simulink model "Model_IEEE_39Bus_GFM_80pct"  (R2024b)
settings: Solver=FixedStepAuto  StartTime=0  StopTime=5  FixedStep=Ts  RelTol=1e-3
values from neighbouring files (symbols this model uses):
  ApparatusDiscreDamping =     [Data_IEEE_39Bus_GFM_100pct.mat]    (also in Data_IEEE_39Bus_GFM_20pct.mat; Data_IEEE_39Bus_GFM_40pct.mat; Data_IEEE_39Bus_GFM_60pct.mat; Data_IEEE_39Bus_GFM_80pct.mat)
  ApparatusPara =     [Data_IEEE_39Bus_GFM_100pct.mat]    (also in Data_IEEE_39Bus_GFM_20pct.mat; Data_IEEE_39Bus_GFM_40pct.mat; Data_IEEE_39Bus_GFM_60pct.mat; Data_IEEE_39Bus_GFM_80pct.mat)
  ApparatusPowerFlow =     [Data_IEEE_39Bus_GFM_100pct.mat]    (also in Data_IEEE_39Bus_GFM_20pct.mat; Data_IEEE_39Bus_GFM_40pct.mat; Data_IEEE_39Bus_GFM_60pct.mat; Data_IEEE_39Bus_GFM_80pct.mat)
  ApparatusType =     [Data_IEEE_39Bus_GFM_100pct.mat]    (also in Data_IEEE_39Bus_GFM_20pct.mat; Data_IEEE_39Bus_GFM_40pct.mat; Data_IEEE_39Bus_GFM_60pct.mat; Data_IEEE_39Bus_GFM_80pct.mat)
  Fbase = 60    [Data_IEEE_39Bus_GFM_100pct.mat]    (also in Data_IEEE_39Bus_GFM_20pct.mat; Data_IEEE_39Bus_GFM_40pct.mat; Data_IEEE_39Bus_GFM_60pct.mat; Data_IEEE_39Bus_GFM_80pct.mat)
  OtherInputs =     [Data_IEEE_39Bus_GFM_100pct.mat]    (also in Data_IEEE_39Bus_GFM_20pct.mat; Data_IEEE_39Bus_GFM_40pct.mat; Data_IEEE_39Bus_GFM_60pct.mat; Data_IEEE_39Bus_GFM_80pct.mat)
  Sbase = 1    [Data_IEEE_39Bus_GFM_100pct.mat]    (also in Data_IEEE_39Bus_GFM_20pct.mat; Data_IEEE_39Bus_GFM_40pct.mat; Data_IEEE_39Bus_GFM_60pct.mat; Data_IEEE_39Bus_GFM_80pct.mat)
  Ts = 3.33333333333e-05    [Data_IEEE_39Bus_GFM_100pct.mat]    (also in Data_IEEE_39Bus_GFM_20pct.mat; Data_IEEE_39Bus_GFM_40pct.mat; Data_IEEE_39Bus_GFM_60pct.mat; Data_IEEE_39Bus_GFM_80pct.mat)
  Vbase = 1    [Data_IEEE_39Bus_GFM_100pct.mat]    (also in Data_IEEE_39Bus_GFM_20pct.mat; Data_IEEE_39Bus_GFM_40pct.mat; Data_IEEE_39Bus_GFM_60pct.mat; Data_IEEE_39Bus_GFM_80pct.mat)
  Wbase = 376.991118431    [Data_IEEE_39Bus_GFM_100pct.mat]    (also in Data_IEEE_39Bus_GFM_20pct.mat; Data_IEEE_39Bus_GFM_40pct.mat; Data_IEEE_39Bus_GFM_60pct.mat; Data_IEEE_39Bus_GFM_80pct.mat)
  x_e =     [Data_IEEE_39Bus_GFM_100pct.mat]    (also in Data_IEEE_39Bus_GFM_20pct.mat; Data_IEEE_39Bus_GFM_40pct.mat; Data_IEEE_39Bus_GFM_60pct.mat; Data_IEEE_39Bus_GFM_80pct.mat)
  Ybase = 1    [Data_IEEE_39Bus_GFM_100pct.mat]    (also in Data_IEEE_39Bus_GFM_20pct.mat; Data_IEEE_39Bus_GFM_40pct.mat; Data_IEEE_39Bus_GFM_60pct.mat; Data_IEEE_39Bus_GFM_80pct.mat)
  Zbase = 1    [Data_IEEE_39Bus_GFM_100pct.mat]    (also in Data_IEEE_39Bus_GFM_20pct.mat; Data_IEEE_39Bus_GFM_40pct.mat; Data_IEEE_39Bus_GFM_60pct.mat; Data_IEEE_39Bus_GFM_80pct.mat)
libraries: SimplusGT x49, spsThreePhaseSeriesRLCBranchLib x46, spsGroundLib x41, spsThreePhaseParallelRLCBranchLib x31, spsThreePhaseTransformerTwoWindingsLib x11, spspowerguiLib x1
settings Model: Creator=皮蛋蛋挞  LastModifiedBy=皮蛋蛋挞

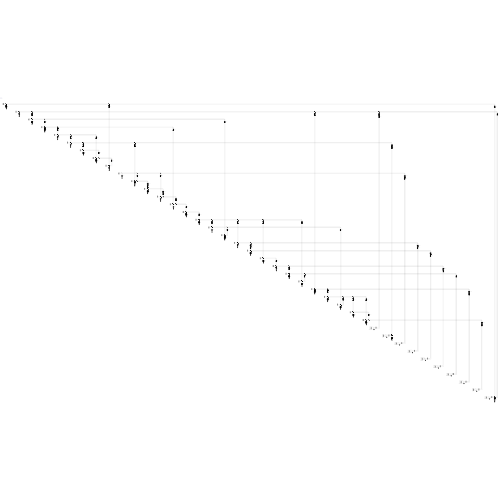
[thumbnail: Simulink's stored preview of the top-level diagram]
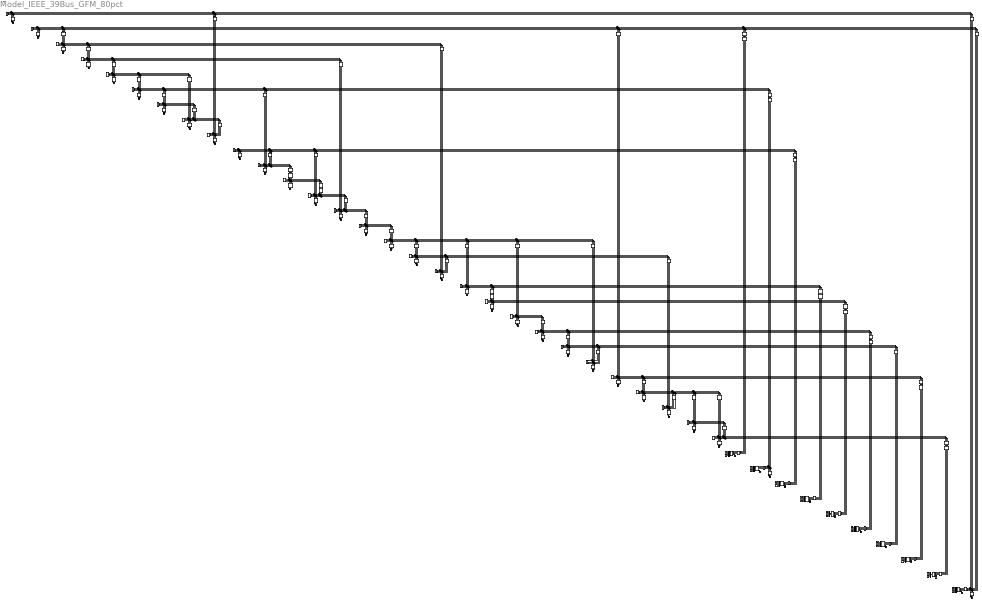
== system Model_IEEE_39Bus_GFM_80pct ==
  B-GND{1,4,9,12,15,18,22,24,26..27,31,33,35,37,39,41,46,49..50,53,55,57,60,63..64,67,71..72,74,76..77} (31 alike) : spsGroundLib/Ground  LConnTagsString=a
  Branch1-1 : spsThreePhaseParallelRLCBranchLib/Three-Phase Parallel RLC Branch  LConnTagsString=A|B|C  RConnTagsString=A|B|C  BranchType=RLC  Resistance=(0.096096)*Zbase  Inductance=(0.42436)*Zbase/Wbase  Capacitance=(0.975)*Ybase/Wbase  Measurements=None
  Branch1-39 : spsThreePhaseSeriesRLCBranchLib/Three-Phase Series RLC Branch  LConnTagsString=A|B|C  RConnTagsString=A|B|C  BranchType=RL  Resistance=(0.001)*Zbase  Inductance=(0.025)*Zbase/Wbase  Capacitance=1e-6  Measurements=None
  Branch1-9 : spsThreePhaseSeriesRLCBranchLib/Three-Phase Series RLC Branch  LConnTagsString=A|B|C  RConnTagsString=A|B|C  BranchType=RL  Resistance=(0.001)*Zbase  Inductance=(0.025)*Zbase/Wbase  Capacitance=1e-6  Measurements=None
  Branch10-10 : spsThreePhaseParallelRLCBranchLib/Three-Phase Parallel RLC Branch  LConnTagsString=A|B|C  RConnTagsString=A|B|C  BranchType=C  Resistance=(Inf)*Zbase  Inductance=(Inf)*Zbase/Wbase  Capacitance=(0.0729)*Ybase/Wbase  Measurements=None
  Branch10-11 : spsThreePhaseSeriesRLCBranchLib/Three-Phase Series RLC Branch  LConnTagsString=A|B|C  RConnTagsString=A|B|C  BranchType=RL  Resistance=(0.0004)*Zbase  Inductance=(0.0043)*Zbase/Wbase  Capacitance=1e-6  Measurements=None
  Branch10-13 : spsThreePhaseSeriesRLCBranchLib/Three-Phase Series RLC Branch  LConnTagsString=A|B|C  RConnTagsString=A|B|C  BranchType=RL  Resistance=(0.0004)*Zbase  Inductance=(0.0043)*Zbase/Wbase  Capacitance=1e-6  Measurements=None
  Branch10-32 : spsThreePhaseSeriesRLCBranchLib/Three-Phase Series RLC Branch  LConnTagsString=A|B|C  RConnTagsString=A|B|C  BranchType=RL  Resistance=(0.001)*Zbase  Inductance=(0.02)*Zbase/Wbase  Capacitance=1e-6  Measurements=None
  Branch11-11 : spsThreePhaseParallelRLCBranchLib/Three-Phase Parallel RLC Branch  LConnTagsString=A|B|C  RConnTagsString=A|B|C  BranchType=C  Resistance=(Inf)*Zbase  Inductance=(Inf)*Zbase/Wbase  Capacitance=(0.1059)*Ybase/Wbase  Measurements=None
  Branch11-12 : spsThreePhaseSeriesRLCBranchLib/Three-Phase Series RLC Branch  LConnTagsString=A|B|C  RConnTagsString=A|B|C  BranchType=RL  Resistance=(0.0016193)*Zbase  Inductance=(0.044024)*Zbase/Wbase  Capacitance=1e-6  Measurements=None
  Branch12-12 : spsThreePhaseParallelRLCBranchLib/Three-Phase Parallel RLC Branch  LConnTagsString=A|B|C  RConnTagsString=A|B|C  BranchType=RL  Resistance=(13.5473)*Zbase  Inductance=(1.1546)*Zbase/Wbase  Capacitance=(0)*Ybase/Wbase  Measurements=None
  Branch12-13 : spsThreePhaseSeriesRLCBranchLib/Three-Phase Series RLC Branch  LConnTagsString=A|B|C  RConnTagsString=A|B|C  BranchType=RL  Resistance=(0.0016)*Zbase  Inductance=(0.0435)*Zbase/Wbase  Capacitance=1e-6  Measurements=None
  Branch13-13 : spsThreePhaseParallelRLCBranchLib/Three-Phase Parallel RLC Branch  LConnTagsString=A|B|C  RConnTagsString=A|B|C  BranchType=C  Resistance=(Inf)*Zbase  Inductance=(Inf)*Zbase/Wbase  Capacitance=(0.1226)*Ybase/Wbase  Measurements=None
  Branch13-14 : spsThreePhaseSeriesRLCBranchLib/Three-Phase Series RLC Branch  LConnTagsString=A|B|C  RConnTagsString=A|B|C  BranchType=RL  Resistance=(0.0009)*Zbase  Inductance=(0.0101)*Zbase/Wbase  Capacitance=1e-6  Measurements=None
  Branch14-14 : spsThreePhaseParallelRLCBranchLib/Three-Phase Parallel RLC Branch  LConnTagsString=A|B|C  RConnTagsString=A|B|C  BranchType=C  Resistance=(Inf)*Zbase  Inductance=(Inf)*Zbase/Wbase  Capacitance=(0.33825)*Ybase/Wbase  Measurements=None
  Branch14-15 : spsThreePhaseSeriesRLCBranchLib/Three-Phase Series RLC Branch  LConnTagsString=A|B|C  RConnTagsString=A|B|C  BranchType=RL  Resistance=(0.0018)*Zbase  Inductance=(0.0217)*Zbase/Wbase  Capacitance=1e-6  Measurements=None
  Branch15-15 : spsThreePhaseParallelRLCBranchLib/Three-Phase Parallel RLC Branch  LConnTagsString=A|B|C  RConnTagsString=A|B|C  BranchType=RLC  Resistance=(0.32386)*Zbase  Inductance=(0.67736)*Zbase/Wbase  Capacitance=(0.2685)*Ybase/Wbase  Measurements=None
  Branch15-16 : spsThreePhaseSeriesRLCBranchLib/Three-Phase Series RLC Branch  LConnTagsString=A|B|C  RConnTagsString=A|B|C  BranchType=RL  Resistance=(0.0009)*Zbase  Inductance=(0.0094)*Zbase/Wbase  Capacitance=1e-6  Measurements=None
  Branch16-16 : spsThreePhaseParallelRLCBranchLib/Three-Phase Parallel RLC Branch  LConnTagsString=A|B|C  RConnTagsString=A|B|C  BranchType=RLC  Resistance=(0.3242)*Zbase  Inductance=(3.3023)*Zbase/Wbase  Capacitance=(0.466)*Ybase/Wbase  Measurements=None
  Branch16-17 : spsThreePhaseSeriesRLCBranchLib/Three-Phase Series RLC Branch  LConnTagsString=A|B|C  RConnTagsString=A|B|C  BranchType=RL  Resistance=(0.0007)*Zbase  Inductance=(0.0089)*Zbase/Wbase  Capacitance=1e-6  Measurements=None
  Branch16-19 : spsThreePhaseSeriesRLCBranchLib/Three-Phase Series RLC Branch  LConnTagsString=A|B|C  RConnTagsString=A|B|C  BranchType=RL  Resistance=(0.0016)*Zbase  Inductance=(0.0195)*Zbase/Wbase  Capacitance=1e-6  Measurements=None
  Branch16-21 : spsThreePhaseSeriesRLCBranchLib/Three-Phase Series RLC Branch  LConnTagsString=A|B|C  RConnTagsString=A|B|C  BranchType=RL  Resistance=(0.0008)*Zbase  Inductance=(0.0135)*Zbase/Wbase  Capacitance=1e-6  Measurements=None
  Branch16-24 : spsThreePhaseSeriesRLCBranchLib/Three-Phase Series RLC Branch  LConnTagsString=A|B|C  RConnTagsString=A|B|C  BranchType=RL  Resistance=(0.0003)*Zbase  Inductance=(0.0059)*Zbase/Wbase  Capacitance=1e-6  Measurements=None
  Branch17-17 : spsThreePhaseParallelRLCBranchLib/Three-Phase Parallel RLC Branch  LConnTagsString=A|B|C  RConnTagsString=A|B|C  BranchType=C  Resistance=(Inf)*Zbase  Inductance=(Inf)*Zbase/Wbase  Capacitance=(0.29385)*Ybase/Wbase  Measurements=None
  Branch17-18 : spsThreePhaseSeriesRLCBranchLib/Three-Phase Series RLC Branch  LConnTagsString=A|B|C  RConnTagsString=A|B|C  BranchType=RL  Resistance=(0.0007)*Zbase  Inductance=(0.0082)*Zbase/Wbase  Capacitance=1e-6  Measurements=None
  Branch17-27 : spsThreePhaseSeriesRLCBranchLib/Three-Phase Series RLC Branch  LConnTagsString=A|B|C  RConnTagsString=A|B|C  BranchType=RL  Resistance=(0.0013)*Zbase  Inductance=(0.0173)*Zbase/Wbase  Capacitance=1e-6  Measurements=None
  Branch18-18 : spsThreePhaseParallelRLCBranchLib/Three-Phase Parallel RLC Branch  LConnTagsString=A|B|C  RConnTagsString=A|B|C  BranchType=RLC  Resistance=(0.6754)*Zbase  Inductance=(3.5571)*Zbase/Wbase  Capacitance=(0.17285)*Ybase/Wbase  Measurements=None
  Branch19-19 : spsThreePhaseParallelRLCBranchLib/Three-Phase Parallel RLC Branch  LConnTagsString=A|B|C  RConnTagsString=A|B|C  BranchType=C  Resistance=(Inf)*Zbase  Inductance=(Inf)*Zbase/Wbase  Capacitance=(0.152)*Ybase/Wbase  Measurements=None
  Branch19-20 : spsThreePhaseSeriesRLCBranchLib/Three-Phase Series RLC Branch  LConnTagsString=A|B|C  RConnTagsString=A|B|C  BranchType=RL  Resistance=(0.0007)*Zbase  Inductance=(0.0138)*Zbase/Wbase  Capacitance=1e-6  Measurements=None
  Branch19-33 : spsThreePhaseSeriesRLCBranchLib/Three-Phase Series RLC Branch  LConnTagsString=A|B|C  RConnTagsString=A|B|C  BranchType=RL  Resistance=(0.0007)*Zbase  Inductance=(0.0142)*Zbase/Wbase  Capacitance=1e-6  Measurements=None
  Branch2-2 : spsThreePhaseParallelRLCBranchLib/Three-Phase Parallel RLC Branch  LConnTagsString=A|B|C  RConnTagsString=A|B|C  BranchType=C  Resistance=(Inf)*Zbase  Inductance=(Inf)*Zbase/Wbase  Capacitance=(0.55095)*Ybase/Wbase  Measurements=None
  Branch2-25 : spsThreePhaseSeriesRLCBranchLib/Three-Phase Series RLC Branch  LConnTagsString=A|B|C  RConnTagsString=A|B|C  BranchType=RL  Resistance=(0.007)*Zbase  Inductance=(0.0086)*Zbase/Wbase  Capacitance=1e-6  Measurements=None
  Branch2-3 : spsThreePhaseSeriesRLCBranchLib/Three-Phase Series RLC Branch  LConnTagsString=A|B|C  RConnTagsString=A|B|C  BranchType=RL  Resistance=(0.0013)*Zbase  Inductance=(0.0151)*Zbase/Wbase  Capacitance=1e-6  Measurements=None
  Branch2-30 : spsThreePhaseSeriesRLCBranchLib/Three-Phase Series RLC Branch  LConnTagsString=A|B|C  RConnTagsString=A|B|C  BranchType=RL  Resistance=(0.001)*Zbase  Inductance=(0.0181)*Zbase/Wbase  Capacitance=1e-6  Measurements=None
  Branch2-39 : spsThreePhaseSeriesRLCBranchLib/Three-Phase Series RLC Branch  LConnTagsString=A|B|C  RConnTagsString=A|B|C  BranchType=RL  Resistance=(0.0035)*Zbase  Inductance=(0.0411)*Zbase/Wbase  Capacitance=1e-6  Measurements=None
  Branch20-20 : spsThreePhaseParallelRLCBranchLib/Three-Phase Parallel RLC Branch  LConnTagsString=A|B|C  RConnTagsString=A|B|C  BranchType=RL  Resistance=(0.1565)*Zbase  Inductance=(0.9542)*Zbase/Wbase  Capacitance=(0)*Ybase/Wbase  Measurements=None
  Branch20-34 : spsThreePhaseSeriesRLCBranchLib/Three-Phase Series RLC Branch  LConnTagsString=A|B|C  RConnTagsString=A|B|C  BranchType=RL  Resistance=(0.0009)*Zbase  Inductance=(0.018)*Zbase/Wbase  Capacitance=1e-6  Measurements=None
  Branch21-21 : spsThreePhaseParallelRLCBranchLib/Three-Phase Parallel RLC Branch  LConnTagsString=A|B|C  RConnTagsString=A|B|C  BranchType=RLC  Resistance=(0.38793)*Zbase  Inductance=(0.92428)*Zbase/Wbase  Capacitance=(0.25565)*Ybase/Wbase  Measurements=None
  Branch21-22 : spsThreePhaseSeriesRLCBranchLib/Three-Phase Series RLC Branch  LConnTagsString=A|B|C  RConnTagsString=A|B|C  BranchType=RL  Resistance=(0.0008)*Zbase  Inductance=(0.014)*Zbase/Wbase  Capacitance=1e-6  Measurements=None
  Branch22-22 : spsThreePhaseParallelRLCBranchLib/Three-Phase Parallel RLC Branch  LConnTagsString=A|B|C  RConnTagsString=A|B|C  BranchType=C  Resistance=(Inf)*Zbase  Inductance=(Inf)*Zbase/Wbase  Capacitance=(0.22055)*Ybase/Wbase  Measurements=None
  Branch22-23 : spsThreePhaseSeriesRLCBranchLib/Three-Phase Series RLC Branch  LConnTagsString=A|B|C  RConnTagsString=A|B|C  BranchType=RL  Resistance=(0.0006)*Zbase  Inductance=(0.0096)*Zbase/Wbase  Capacitance=1e-6  Measurements=None
  Branch22-35 : spsThreePhaseSeriesRLCBranchLib/Three-Phase Series RLC Branch  LConnTagsString=A|B|C  RConnTagsString=A|B|C  BranchType=RL  Resistance=(0.001)*Zbase  Inductance=(0.0143)*Zbase/Wbase  Capacitance=1e-6  Measurements=None
  Branch23-23 : spsThreePhaseParallelRLCBranchLib/Three-Phase Parallel RLC Branch  LConnTagsString=A|B|C  RConnTagsString=A|B|C  BranchType=RLC  Resistance=(0.43976)*Zbase  Inductance=(1.2865)*Zbase/Wbase  Capacitance=(0.2728)*Ybase/Wbase  Measurements=None
  Branch23-24 : spsThreePhaseSeriesRLCBranchLib/Three-Phase Series RLC Branch  LConnTagsString=A|B|C  RConnTagsString=A|B|C  BranchType=RL  Resistance=(0.0022)*Zbase  Inductance=(0.035)*Zbase/Wbase  Capacitance=1e-6  Measurements=None
  Branch23-36 : spsThreePhaseSeriesRLCBranchLib/Three-Phase Series RLC Branch  LConnTagsString=A|B|C  RConnTagsString=A|B|C  BranchType=RL  Resistance=(0.0005)*Zbase  Inductance=(0.0272)*Zbase/Wbase  Capacitance=1e-6  Measurements=None
  Branch24-24 : spsThreePhaseParallelRLCBranchLib/Three-Phase Parallel RLC Branch  LConnTagsString=A|B|C  RConnTagsString=A|B|C  BranchType=RC  Resistance=(0.3491)*Zbase  Inductance=(Inf)*Zbase/Wbase  Capacitance=(1.0685)*Ybase/Wbase  Measurements=None
  Branch25-25 : spsThreePhaseParallelRLCBranchLib/Three-Phase Parallel RLC Branch  LConnTagsString=A|B|C  RConnTagsString=A|B|C  BranchType=RLC  Resistance=(0.49976)*Zbase  Inductance=(2.3717)*Zbase/Wbase  Capacitance=(0.3295)*Ybase/Wbase  Measurements=None
  Branch25-26 : spsThreePhaseSeriesRLCBranchLib/Three-Phase Series RLC Branch  LConnTagsString=A|B|C  RConnTagsString=A|B|C  BranchType=RL  Resistance=(0.0032)*Zbase  Inductance=(0.0323)*Zbase/Wbase  Capacitance=1e-6  Measurements=None
  Branch25-37 : spsThreePhaseSeriesRLCBranchLib/Three-Phase Series RLC Branch  LConnTagsString=A|B|C  RConnTagsString=A|B|C  BranchType=RL  Resistance=(0.0006)*Zbase  Inductance=(0.0232)*Zbase/Wbase  Capacitance=1e-6  Measurements=None
  Branch26-26 : spsThreePhaseParallelRLCBranchLib/Three-Phase Parallel RLC Branch  LConnTagsString=A|B|C  RConnTagsString=A|B|C  BranchType=RLC  Resistance=(0.7975)*Zbase  Inductance=(6.5207)*Zbase/Wbase  Capacitance=(1.2809)*Ybase/Wbase  Measurements=None
  Branch26-27 : spsThreePhaseSeriesRLCBranchLib/Three-Phase Series RLC Branch  LConnTagsString=A|B|C  RConnTagsString=A|B|C  BranchType=RL  Resistance=(0.0014)*Zbase  Inductance=(0.0147)*Zbase/Wbase  Capacitance=1e-6  Measurements=None
  Branch26-28 : spsThreePhaseSeriesRLCBranchLib/Three-Phase Series RLC Branch  LConnTagsString=A|B|C  RConnTagsString=A|B|C  BranchType=RL  Resistance=(0.0043)*Zbase  Inductance=(0.0474)*Zbase/Wbase  Capacitance=1e-6  Measurements=None
  Branch26-29 : spsThreePhaseSeriesRLCBranchLib/Three-Phase Series RLC Branch  LConnTagsString=A|B|C  RConnTagsString=A|B|C  BranchType=RL  Resistance=(0.0057)*Zbase  Inductance=(0.0625)*Zbase/Wbase  Capacitance=1e-6  Measurements=None
  Branch27-27 : spsThreePhaseParallelRLCBranchLib/Three-Phase Parallel RLC Branch  LConnTagsString=A|B|C  RConnTagsString=A|B|C  BranchType=RLC  Resistance=(0.38408)*Zbase  Inductance=(1.4295)*Zbase/Wbase  Capacitance=(0.2806)*Ybase/Wbase  Measurements=None
  Branch28-28 : spsThreePhaseParallelRLCBranchLib/Three-Phase Parallel RLC Branch  LConnTagsString=A|B|C  RConnTagsString=A|B|C  BranchType=RLC  Resistance=(0.53574)*Zbase  Inductance=(3.9986)*Zbase/Wbase  Capacitance=(0.5146)*Ybase/Wbase  Measurements=None
  Branch28-29 : spsThreePhaseSeriesRLCBranchLib/Three-Phase Series RLC Branch  LConnTagsString=A|B|C  RConnTagsString=A|B|C  BranchType=RL  Resistance=(0.0014)*Zbase  Inductance=(0.0151)*Zbase/Wbase  Capacitance=1e-6  Measurements=None
  Branch29-29 : spsThreePhaseParallelRLCBranchLib/Three-Phase Parallel RLC Branch  LConnTagsString=A|B|C  RConnTagsString=A|B|C  BranchType=RLC  Resistance=(0.38905)*Zbase  Inductance=(4.1003)*Zbase/Wbase  Capacitance=(0.639)*Ybase/Wbase  Measurements=None
  Branch29-38 : spsThreePhaseSeriesRLCBranchLib/Three-Phase Series RLC Branch  LConnTagsString=A|B|C  RConnTagsString=A|B|C  BranchType=RL  Resistance=(0.0008)*Zbase  Inductance=(0.0156)*Zbase/Wbase  Capacitance=1e-6  Measurements=None
  Branch3-18 : spsThreePhaseSeriesRLCBranchLib/Three-Phase Series RLC Branch  LConnTagsString=A|B|C  RConnTagsString=A|B|C  BranchType=RL  Resistance=(0.0011)*Zbase  Inductance=(0.0133)*Zbase/Wbase  Capacitance=1e-6  Measurements=None
  Branch3-3 : spsThreePhaseParallelRLCBranchLib/Three-Phase Parallel RLC Branch  LConnTagsString=A|B|C  RConnTagsString=A|B|C  BranchType=RLC  Resistance=(0.33154)*Zbase  Inductance=(44.4819)*Zbase/Wbase  Capacitance=(0.3462)*Ybase/Wbase  Measurements=None
  Branch3-4 : spsThreePhaseSeriesRLCBranchLib/Three-Phase Series RLC Branch  LConnTagsString=A|B|C  RConnTagsString=A|B|C  BranchType=RL  Resistance=(0.0013)*Zbase  Inductance=(0.0213)*Zbase/Wbase  Capacitance=1e-6  Measurements=None
  Branch31-31 : spsThreePhaseParallelRLCBranchLib/Three-Phase Parallel RLC Branch  LConnTagsString=A|B|C  RConnTagsString=A|B|C  BranchType=RL  Resistance=(10.4818)*Zbase  Inductance=(20.9636)*Zbase/Wbase  Capacitance=(0)*Ybase/Wbase  Measurements=None
  Branch39-39 : spsThreePhaseParallelRLCBranchLib/Three-Phase Parallel RLC Branch  LConnTagsString=A|B|C  RConnTagsString=A|B|C  BranchType=C  Resistance=(Inf)*Zbase  Inductance=(Inf)*Zbase/Wbase  Capacitance=(0.72435)*Ybase/Wbase  Measurements=None
  Branch4-14 : spsThreePhaseSeriesRLCBranchLib/Three-Phase Series RLC Branch  LConnTagsString=A|B|C  RConnTagsString=A|B|C  BranchType=RL  Resistance=(0.0008)*Zbase  Inductance=(0.0129)*Zbase/Wbase  Capacitance=1e-6  Measurements=None
  Branch4-4 : spsThreePhaseParallelRLCBranchLib/Three-Phase Parallel RLC Branch  LConnTagsString=A|B|C  RConnTagsString=A|B|C  BranchType=RLC  Resistance=(0.2048)*Zbase  Inductance=(0.55653)*Zbase/Wbase  Capacitance=(0.2469)*Ybase/Wbase  Measurements=None
  Branch4-5 : spsThreePhaseSeriesRLCBranchLib/Three-Phase Series RLC Branch  LConnTagsString=A|B|C  RConnTagsString=A|B|C  BranchType=RL  Resistance=(0.0008)*Zbase  Inductance=(0.0128)*Zbase/Wbase  Capacitance=1e-6  Measurements=None
  Branch5-5 : spsThreePhaseParallelRLCBranchLib/Three-Phase Parallel RLC Branch  LConnTagsString=A|B|C  RConnTagsString=A|B|C  BranchType=C  Resistance=(Inf)*Zbase  Inductance=(Inf)*Zbase/Wbase  Capacitance=(0.1626)*Ybase/Wbase  Measurements=None
  Branch5-6 : spsThreePhaseSeriesRLCBranchLib/Three-Phase Series RLC Branch  LConnTagsString=A|B|C  RConnTagsString=A|B|C  BranchType=RL  Resistance=(0.0002)*Zbase  Inductance=(0.0026)*Zbase/Wbase  Capacitance=1e-6  Measurements=None
  Branch5-8 : spsThreePhaseSeriesRLCBranchLib/Three-Phase Series RLC Branch  LConnTagsString=A|B|C  RConnTagsString=A|B|C  BranchType=RL  Resistance=(0.0008)*Zbase  Inductance=(0.0112)*Zbase/Wbase  Capacitance=1e-6  Measurements=None
  Branch6-11 : spsThreePhaseSeriesRLCBranchLib/Three-Phase Series RLC Branch  LConnTagsString=A|B|C  RConnTagsString=A|B|C  BranchType=RL  Resistance=(0.0007)*Zbase  Inductance=(0.0082)*Zbase/Wbase  Capacitance=1e-6  Measurements=None
  Branch6-31 : spsThreePhaseSeriesRLCBranchLib/Three-Phase Series RLC Branch  LConnTagsString=A|B|C  RConnTagsString=A|B|C  BranchType=RL  Resistance=(0.00081)*Zbase  Inductance=(0.02025)*Zbase/Wbase  Capacitance=1e-6  Measurements=None
  Branch6-6 : spsThreePhaseParallelRLCBranchLib/Three-Phase Parallel RLC Branch  LConnTagsString=A|B|C  RConnTagsString=A|B|C  BranchType=C  Resistance=(Inf)*Zbase  Inductance=(Inf)*Zbase/Wbase  Capacitance=(0.14765)*Ybase/Wbase  Measurements=None
  Branch6-7 : spsThreePhaseSeriesRLCBranchLib/Three-Phase Series RLC Branch  LConnTagsString=A|B|C  RConnTagsString=A|B|C  BranchType=RL  Resistance=(0.0006)*Zbase  Inductance=(0.0092)*Zbase/Wbase  Capacitance=1e-6  Measurements=None
  Branch7-7 : spsThreePhaseParallelRLCBranchLib/Three-Phase Parallel RLC Branch  LConnTagsString=A|B|C  RConnTagsString=A|B|C  BranchType=RLC  Resistance=(0.43604)*Zbase  Inductance=(1.2137)*Zbase/Wbase  Capacitance=(0.0955)*Ybase/Wbase  Measurements=None
  Branch7-8 : spsThreePhaseSeriesRLCBranchLib/Three-Phase Series RLC Branch  LConnTagsString=A|B|C  RConnTagsString=A|B|C  BranchType=RL  Resistance=(0.0004)*Zbase  Inductance=(0.0046)*Zbase/Wbase  Capacitance=1e-6  Measurements=None
  Branch8-8 : spsThreePhaseParallelRLCBranchLib/Three-Phase Parallel RLC Branch  LConnTagsString=A|B|C  RConnTagsString=A|B|C  BranchType=RLC  Resistance=(0.1947)*Zbase  Inductance=(0.57745)*Zbase/Wbase  Capacitance=(0.303)*Ybase/Wbase  Measurements=None
  Branch8-9 : spsThreePhaseSeriesRLCBranchLib/Three-Phase Series RLC Branch  LConnTagsString=A|B|C  RConnTagsString=A|B|C  BranchType=RL  Resistance=(0.0023)*Zbase  Inductance=(0.0363)*Zbase/Wbase  Capacitance=1e-6  Measurements=None
  Branch9-9 : spsThreePhaseParallelRLCBranchLib/Three-Phase Parallel RLC Branch  LConnTagsString=A|B|C  RConnTagsString=A|B|C  BranchType=C  Resistance=(Inf)*Zbase  Inductance=(Inf)*Zbase/Wbase  Capacitance=(0.7902)*Ybase/Wbase  Measurements=None
  Bus{1..39} (39 alike) : SimplusGT/Three-Phase Bus  Vbase=1  Sbase=1
  D-GND{30..39} (10 alike) : spsGroundLib/Ground  LConnTagsString=a
  D-Scope{30..39} (10 alike) : Scope  NumInputPorts=7
  DS-Bus{30..39} (10 alike) : BusSelector  OutputSignals=v_dq,i_dq,v_abc,i_abc,w,theta,pq
  Transformer10-32 : spsThreePhaseTransformerTwoWindingsLib/Three-Phase Transformer (Two Windings)  Winding1Connection=Yg  Winding2Connection=Yg  CoreType=Three single-phase transformers  SetSaturation=off  Hysteresis=off  DataFile='hysteresis'  SetInitialFlux=off  Measurements=None  UNITS=pu  NominalPower=[Sbase, Fbase]  Winding1=[1.07*Vbase, 0, 0]  Winding2=[Vbase, 0, 0]  Rm=1e4  Lm=1e4  L0=0.5  Saturation=[ 0,0 ; 0.0024,1.2 ; 1.0,1.52 ]  InitialFluxes=[ 0.8 , -0.8 , 0.7 ]  BreakLoop=off  DiscreteSolver=Trapezoidal iterative  DataType=off  TransfoNumber=1
  Transformer11-12 : spsThreePhaseTransformerTwoWindingsLib/Three-Phase Transformer (Two Windings)  Winding1Connection=Yg  Winding2Connection=Yg  CoreType=Three single-phase transformers  SetSaturation=off  Hysteresis=off  DataFile='hysteresis'  SetInitialFlux=off  Measurements=None  UNITS=pu  NominalPower=[Sbase, Fbase]  Winding1=[0.99404*Vbase, 0, 0]  Winding2=[Vbase, 0, 0]  Rm=1e4  Lm=1e4  L0=0.5  Saturation=[ 0,0 ; 0.0024,1.2 ; 1.0,1.52 ]  InitialFluxes=[ 0.8 , -0.8 , 0.7 ]  BreakLoop=off  DiscreteSolver=Trapezoidal iterative  DataType=off  TransfoNumber=1
  Transformer12-13 : spsThreePhaseTransformerTwoWindingsLib/Three-Phase Transformer (Two Windings)  Winding1Connection=Yg  Winding2Connection=Yg  CoreType=Three single-phase transformers  SetSaturation=off  Hysteresis=off  DataFile='hysteresis'  SetInitialFlux=off  Measurements=None  UNITS=pu  NominalPower=[Sbase, Fbase]  Winding1=[1.006*Vbase, 0, 0]  Winding2=[Vbase, 0, 0]  Rm=1e4  Lm=1e4  L0=0.5  Saturation=[ 0,0 ; 0.0024,1.2 ; 1.0,1.52 ]  InitialFluxes=[ 0.8 , -0.8 , 0.7 ]  BreakLoop=off  DiscreteSolver=Trapezoidal iterative  DataType=off  TransfoNumber=1
  Transformer19-20 : spsThreePhaseTransformerTwoWindingsLib/Three-Phase Transformer (Two Windings)  Winding1Connection=Yg  Winding2Connection=Yg  CoreType=Three single-phase transformers  SetSaturation=off  Hysteresis=off  DataFile='hysteresis'  SetInitialFlux=off  Measurements=None  UNITS=pu  NominalPower=[Sbase, Fbase]  Winding1=[1.06*Vbase, 0, 0]  Winding2=[Vbase, 0, 0]  Rm=1e4  Lm=1e4  L0=0.5  Saturation=[ 0,0 ; 0.0024,1.2 ; 1.0,1.52 ]  InitialFluxes=[ 0.8 , -0.8 , 0.7 ]  BreakLoop=off  DiscreteSolver=Trapezoidal iterative  DataType=off  TransfoNumber=1
  Transformer19-33 : spsThreePhaseTransformerTwoWindingsLib/Three-Phase Transformer (Two Windings)  Winding1Connection=Yg  Winding2Connection=Yg  CoreType=Three single-phase transformers  SetSaturation=off  Hysteresis=off  DataFile='hysteresis'  SetInitialFlux=off  Measurements=None  UNITS=pu  NominalPower=[Sbase, Fbase]  Winding1=[1.07*Vbase, 0, 0]  Winding2=[Vbase, 0, 0]  Rm=1e4  Lm=1e4  L0=0.5  Saturation=[ 0,0 ; 0.0024,1.2 ; 1.0,1.52 ]  InitialFluxes=[ 0.8 , -0.8 , 0.7 ]  BreakLoop=off  DiscreteSolver=Trapezoidal iterative  DataType=off  TransfoNumber=1
  Transformer2-30 : spsThreePhaseTransformerTwoWindingsLib/Three-Phase Transformer (Two Windings)  Winding1Connection=Yg  Winding2Connection=Yg  CoreType=Three single-phase transformers  SetSaturation=off  Hysteresis=off  DataFile='hysteresis'  SetInitialFlux=off  Measurements=None  UNITS=pu  NominalPower=[Sbase, Fbase]  Winding1=[1.025*Vbase, 0, 0]  Winding2=[Vbase, 0, 0]  Rm=1e4  Lm=1e4  L0=0.5  Saturation=[ 0,0 ; 0.0024,1.2 ; 1.0,1.52 ]  InitialFluxes=[ 0.8 , -0.8 , 0.7 ]  BreakLoop=off  DiscreteSolver=Trapezoidal iterative  DataType=off  TransfoNumber=1
  Transformer20-34 : spsThreePhaseTransformerTwoWindingsLib/Three-Phase Transformer (Two Windings)  Winding1Connection=Yg  Winding2Connection=Yg  CoreType=Three single-phase transformers  SetSaturation=off  Hysteresis=off  DataFile='hysteresis'  SetInitialFlux=off  Measurements=None  UNITS=pu  NominalPower=[Sbase, Fbase]  Winding1=[1.009*Vbase, 0, 0]  Winding2=[Vbase, 0, 0]  Rm=1e4  Lm=1e4  L0=0.5  Saturation=[ 0,0 ; 0.0024,1.2 ; 1.0,1.52 ]  InitialFluxes=[ 0.8 , -0.8 , 0.7 ]  BreakLoop=off  DiscreteSolver=Trapezoidal iterative  DataType=off  TransfoNumber=1
  Transformer22-35 : spsThreePhaseTransformerTwoWindingsLib/Three-Phase Transformer (Two Windings)  Winding1Connection=Yg  Winding2Connection=Yg  CoreType=Three single-phase transformers  SetSaturation=off  Hysteresis=off  DataFile='hysteresis'  SetInitialFlux=off  Measurements=None  UNITS=pu  NominalPower=[Sbase, Fbase]  Winding1=[1.025*Vbase, 0, 0]  Winding2=[Vbase, 0, 0]  Rm=1e4  Lm=1e4  L0=0.5  Saturation=[ 0,0 ; 0.0024,1.2 ; 1.0,1.52 ]  InitialFluxes=[ 0.8 , -0.8 , 0.7 ]  BreakLoop=off  DiscreteSolver=Trapezoidal iterative  DataType=off  TransfoNumber=1
  Transformer25-37 : spsThreePhaseTransformerTwoWindingsLib/Three-Phase Transformer (Two Windings)  Winding1Connection=Yg  Winding2Connection=Yg  CoreType=Three single-phase transformers  SetSaturation=off  Hysteresis=off  DataFile='hysteresis'  SetInitialFlux=off  Measurements=None  UNITS=pu  NominalPower=[Sbase, Fbase]  Winding1=[1.025*Vbase, 0, 0]  Winding2=[Vbase, 0, 0]  Rm=1e4  Lm=1e4  L0=0.5  Saturation=[ 0,0 ; 0.0024,1.2 ; 1.0,1.52 ]  InitialFluxes=[ 0.8 , -0.8 , 0.7 ]  BreakLoop=off  DiscreteSolver=Trapezoidal iterative  DataType=off  TransfoNumber=1
  Transformer29-38 : spsThreePhaseTransformerTwoWindingsLib/Three-Phase Transformer (Two Windings)  Winding1Connection=Yg  Winding2Connection=Yg  CoreType=Three single-phase transformers  SetSaturation=off  Hysteresis=off  DataFile='hysteresis'  SetInitialFlux=off  Measurements=None  UNITS=pu  NominalPower=[Sbase, Fbase]  Winding1=[1.025*Vbase, 0, 0]  Winding2=[Vbase, 0, 0]  Rm=1e4  Lm=1e4  L0=0.5  Saturation=[ 0,0 ; 0.0024,1.2 ; 1.0,1.52 ]  InitialFluxes=[ 0.8 , -0.8 , 0.7 ]  BreakLoop=off  DiscreteSolver=Trapezoidal iterative  DataType=off  TransfoNumber=1
  Transformer6-31 : spsThreePhaseTransformerTwoWindingsLib/Three-Phase Transformer (Two Windings)  Winding1Connection=Yg  Winding2Connection=Yg  CoreType=Three single-phase transformers  SetSaturation=off  Hysteresis=off  DataFile='hysteresis'  SetInitialFlux=off  Measurements=None  UNITS=pu  NominalPower=[Sbase, Fbase]  Winding1=[1.1111*Vbase, 0, 0]  Winding2=[Vbase, 0, 0]  Rm=1e4  Lm=1e4  L0=0.5  Saturation=[ 0,0 ; 0.0024,1.2 ; 1.0,1.52 ]  InitialFluxes=[ 0.8 , -0.8 , 0.7 ]  BreakLoop=off  DiscreteSolver=Trapezoidal iterative  DataType=off  TransfoNumber=1
  VSI-Droop30 : SimplusGT/Grid-Forming Voltage-Source Inverter (dq-Frame System Object)  Ts=Ts  Sbase=Sbase  Vbase=Vbase  Wbase=Wbase  ApparatusType=ApparatusType{30}  ApparatusPara=ApparatusPara{30}  PowerFlow=ApparatusPowerFlow{30}  x0=x_e{30}  OtherInputs=OtherInputs{30}  DiscreMethod=Hybrid Trapezoidal  EnableInsideModification=off  DiscreDampingFlag=on  DiscreDampingValue=ApparatusDiscreDamping{30}  LinearizationTimes=1  DirectFeedthrough=off
  VSI-Droop31 : SimplusGT/Grid-Forming Voltage-Source Inverter (dq-Frame System Object)  Ts=Ts  Sbase=Sbase  Vbase=Vbase  Wbase=Wbase  ApparatusType=ApparatusType{31}  ApparatusPara=ApparatusPara{31}  PowerFlow=ApparatusPowerFlow{31}  x0=x_e{31}  OtherInputs=OtherInputs{31}  DiscreMethod=Hybrid Trapezoidal  EnableInsideModification=off  DiscreDampingFlag=on  DiscreDampingValue=ApparatusDiscreDamping{31}  LinearizationTimes=1  DirectFeedthrough=off
  VSI-Droop32 : SimplusGT/Grid-Forming Voltage-Source Inverter (dq-Frame System Object)  Ts=Ts  Sbase=Sbase  Vbase=Vbase  Wbase=Wbase  ApparatusType=ApparatusType{32}  ApparatusPara=ApparatusPara{32}  PowerFlow=ApparatusPowerFlow{32}  x0=x_e{32}  OtherInputs=OtherInputs{32}  DiscreMethod=Hybrid Trapezoidal  EnableInsideModification=off  DiscreDampingFlag=on  DiscreDampingValue=ApparatusDiscreDamping{32}  LinearizationTimes=1  DirectFeedthrough=off
  VSI-Droop33 : SimplusGT/Grid-Forming Voltage-Source Inverter (dq-Frame System Object)  Ts=Ts  Sbase=Sbase  Vbase=Vbase  Wbase=Wbase  ApparatusType=ApparatusType{33}  ApparatusPara=ApparatusPara{33}  PowerFlow=ApparatusPowerFlow{33}  x0=x_e{33}  OtherInputs=OtherInputs{33}  DiscreMethod=Hybrid Trapezoidal  EnableInsideModification=off  DiscreDampingFlag=on  DiscreDampingValue=ApparatusDiscreDamping{33}  LinearizationTimes=1  DirectFeedthrough=off
  VSI-Droop34 : SimplusGT/Grid-Forming Voltage-Source Inverter (dq-Frame System Object)  Ts=Ts  Sbase=Sbase  Vbase=Vbase  Wbase=Wbase  ApparatusType=ApparatusType{34}  ApparatusPara=ApparatusPara{34}  PowerFlow=ApparatusPowerFlow{34}  x0=x_e{34}  OtherInputs=OtherInputs{34}  DiscreMethod=Hybrid Trapezoidal  EnableInsideModification=off  DiscreDampingFlag=on  DiscreDampingValue=ApparatusDiscreDamping{34}  LinearizationTimes=1  DirectFeedthrough=off
  VSI-Droop35 : SimplusGT/Grid-Forming Voltage-Source Inverter (dq-Frame System Object)  Ts=Ts  Sbase=Sbase  Vbase=Vbase  Wbase=Wbase  ApparatusType=ApparatusType{35}  ApparatusPara=ApparatusPara{35}  PowerFlow=ApparatusPowerFlow{35}  x0=x_e{35}  OtherInputs=OtherInputs{35}  DiscreMethod=Hybrid Trapezoidal  EnableInsideModification=off  DiscreDampingFlag=on  DiscreDampingValue=ApparatusDiscreDamping{35}  LinearizationTimes=1  DirectFeedthrough=off
  VSI-Droop36 : SimplusGT/Grid-Forming Voltage-Source Inverter (dq-Frame System Object)  Ts=Ts  Sbase=Sbase  Vbase=Vbase  Wbase=Wbase  ApparatusType=ApparatusType{36}  ApparatusPara=ApparatusPara{36}  PowerFlow=ApparatusPowerFlow{36}  x0=x_e{36}  OtherInputs=OtherInputs{36}  DiscreMethod=Hybrid Trapezoidal  EnableInsideModification=off  DiscreDampingFlag=on  DiscreDampingValue=ApparatusDiscreDamping{36}  LinearizationTimes=1  DirectFeedthrough=off
  VSI-Droop37 : SimplusGT/Grid-Forming Voltage-Source Inverter (dq-Frame System Object)  Ts=Ts  Sbase=Sbase  Vbase=Vbase  Wbase=Wbase  ApparatusType=ApparatusType{37}  ApparatusPara=ApparatusPara{37}  PowerFlow=ApparatusPowerFlow{37}  x0=x_e{37}  OtherInputs=OtherInputs{37}  DiscreMethod=Hybrid Trapezoidal  EnableInsideModification=off  DiscreDampingFlag=on  DiscreDampingValue=ApparatusDiscreDamping{37}  LinearizationTimes=1  DirectFeedthrough=off
  VSI-PLL38 : SimplusGT/Grid-Following Voltage-Source Inverter (dq-Frame System Object)  Ts=Ts  Sbase=Sbase  Vbase=Vbase  Wbase=Wbase  ApparatusType=ApparatusType{38}  ApparatusPara=ApparatusPara{38}  PowerFlow=ApparatusPowerFlow{38}  x0=x_e{38}  OtherInputs=OtherInputs{38}  DiscreMethod=Hybrid Trapezoidal  EnableInsideModification=off  DiscreDampingFlag=on  DiscreDampingValue=ApparatusDiscreDamping{38}  LinearizationTimes=1  DirectFeedthrough=off
  VSI-PLL39 : SimplusGT/Grid-Following Voltage-Source Inverter (dq-Frame System Object)  Ts=Ts  Sbase=Sbase  Vbase=Vbase  Wbase=Wbase  ApparatusType=ApparatusType{39}  ApparatusPara=ApparatusPara{39}  PowerFlow=ApparatusPowerFlow{39}  x0=x_e{39}  OtherInputs=OtherInputs{39}  DiscreMethod=Hybrid Trapezoidal  EnableInsideModification=off  DiscreDampingFlag=on  DiscreDampingValue=ApparatusDiscreDamping{39}  LinearizationTimes=1  DirectFeedthrough=off
  powergui : spspowerguiLib/powergui  Priority=1  SimulationMode=Discrete  SampleTime=Ts  frequency=60  Iterations=50  frequencyindice=60  Pbase=100e6  ErrMax=1e-4  UnitsV=kV  UnitsW=MW  buscounter=0  FunctionMessages=off  echomessages=off  EnableUseOfTLC=off  CurrentSourceSwitches=off  DisableSnubberDevices=off  DisableRonSwitches=off  DisableVfSwitches=off  DisplayEquations=off  AutomaticDiscreteSolvers=off  SolverType=Tustin/Backward Euler (TBE)  Interpol=off  ExternalGateDelay=off  methode=off  Ts=100  x0status=blocks  SPID=on  SwTol=0  HookPort=off  NonlinearTolerance=1e-4  nMaxIteration=100  ContinueOnMaxIteration=off  RestoreLinks=warning  ResistiveCurrentMeasurement=off  Frange=[0:2:500]  Ylog=off  Xlog=on  ShowGrid=off  save=off  variable=ZData  structure=0  ZoomFFT=off  StartTime=0.0  cycles=1  DisplayStyle=1  fundamental=60  FreqAxis=off  MaxFrequency=1000  frequencyindicesteady=1  RmsSteady=1  display=off
  wires:
  VSI-Droop30/1 -> DS-Bus30/1
  DS-Bus30/1 -> D-Scope30/1  "<v_dq>"
  DS-Bus30/2 -> D-Scope30/2  "<i_dq>"
  DS-Bus30/3 -> D-Scope30/3  "<v_abc>"
  DS-Bus30/4 -> D-Scope30/4  "<i_abc>"
  DS-Bus30/5 -> D-Scope30/5  "<w>"
  DS-Bus30/6 -> D-Scope30/6  "<theta>"
  DS-Bus30/7 -> D-Scope30/7  "<pq>"
  VSI-Droop31/1 -> DS-Bus31/1
  DS-Bus31/1 -> D-Scope31/1  "<v_dq>"
  DS-Bus31/2 -> D-Scope31/2  "<i_dq>"
  DS-Bus31/3 -> D-Scope31/3  "<v_abc>"
  DS-Bus31/4 -> D-Scope31/4  "<i_abc>"
  DS-Bus31/5 -> D-Scope31/5  "<w>"
  DS-Bus31/6 -> D-Scope31/6  "<theta>"
  DS-Bus31/7 -> D-Scope31/7  "<pq>"
  VSI-Droop32/1 -> DS-Bus32/1
  DS-Bus32/1 -> D-Scope32/1  "<v_dq>"
  DS-Bus32/2 -> D-Scope32/2  "<i_dq>"
  DS-Bus32/3 -> D-Scope32/3  "<v_abc>"
  DS-Bus32/4 -> D-Scope32/4  "<i_abc>"
  DS-Bus32/5 -> D-Scope32/5  "<w>"
  DS-Bus32/6 -> D-Scope32/6  "<theta>"
  DS-Bus32/7 -> D-Scope32/7  "<pq>"
  VSI-Droop33/1 -> DS-Bus33/1
  DS-Bus33/1 -> D-Scope33/1  "<v_dq>"
  DS-Bus33/2 -> D-Scope33/2  "<i_dq>"
  DS-Bus33/3 -> D-Scope33/3  "<v_abc>"
  DS-Bus33/4 -> D-Scope33/4  "<i_abc>"
  DS-Bus33/5 -> D-Scope33/5  "<w>"
  DS-Bus33/6 -> D-Scope33/6  "<theta>"
  DS-Bus33/7 -> D-Scope33/7  "<pq>"
  VSI-Droop34/1 -> DS-Bus34/1
  DS-Bus34/1 -> D-Scope34/1  "<v_dq>"
  DS-Bus34/2 -> D-Scope34/2  "<i_dq>"
  DS-Bus34/3 -> D-Scope34/3  "<v_abc>"
  DS-Bus34/4 -> D-Scope34/4  "<i_abc>"
  DS-Bus34/5 -> D-Scope34/5  "<w>"
  DS-Bus34/6 -> D-Scope34/6  "<theta>"
  DS-Bus34/7 -> D-Scope34/7  "<pq>"
  VSI-Droop35/1 -> DS-Bus35/1
  DS-Bus35/1 -> D-Scope35/1  "<v_dq>"
  DS-Bus35/2 -> D-Scope35/2  "<i_dq>"
  DS-Bus35/3 -> D-Scope35/3  "<v_abc>"
  DS-Bus35/4 -> D-Scope35/4  "<i_abc>"
  DS-Bus35/5 -> D-Scope35/5  "<w>"
  DS-Bus35/6 -> D-Scope35/6  "<theta>"
  DS-Bus35/7 -> D-Scope35/7  "<pq>"
  VSI-Droop36/1 -> DS-Bus36/1
  DS-Bus36/1 -> D-Scope36/1  "<v_dq>"
  DS-Bus36/2 -> D-Scope36/2  "<i_dq>"
  DS-Bus36/3 -> D-Scope36/3  "<v_abc>"
  DS-Bus36/4 -> D-Scope36/4  "<i_abc>"
  DS-Bus36/5 -> D-Scope36/5  "<w>"
  DS-Bus36/6 -> D-Scope36/6  "<theta>"
  DS-Bus36/7 -> D-Scope36/7  "<pq>"
  VSI-Droop37/1 -> DS-Bus37/1
  DS-Bus37/1 -> D-Scope37/1  "<v_dq>"
  DS-Bus37/2 -> D-Scope37/2  "<i_dq>"
  DS-Bus37/3 -> D-Scope37/3  "<v_abc>"
  DS-Bus37/4 -> D-Scope37/4  "<i_abc>"
  DS-Bus37/5 -> D-Scope37/5  "<w>"
  DS-Bus37/6 -> D-Scope37/6  "<theta>"
  DS-Bus37/7 -> D-Scope37/7  "<pq>"
  VSI-PLL38/1 -> DS-Bus38/1
  DS-Bus38/1 -> D-Scope38/1  "<v_dq>"
  DS-Bus38/2 -> D-Scope38/2  "<i_dq>"
  DS-Bus38/3 -> D-Scope38/3  "<v_abc>"
  DS-Bus38/4 -> D-Scope38/4  "<i_abc>"
  DS-Bus38/5 -> D-Scope38/5  "<w>"
  DS-Bus38/6 -> D-Scope38/6  "<theta>"
  DS-Bus38/7 -> D-Scope38/7  "<pq>"
  VSI-PLL39/1 -> DS-Bus39/1
  DS-Bus39/1 -> D-Scope39/1  "<v_dq>"
  DS-Bus39/2 -> D-Scope39/2  "<i_dq>"
  DS-Bus39/3 -> D-Scope39/3  "<v_abc>"
  DS-Bus39/4 -> D-Scope39/4  "<i_abc>"
  DS-Bus39/5 -> D-Scope39/5  "<w>"
  DS-Bus39/6 -> D-Scope39/6  "<theta>"
  DS-Bus39/7 -> D-Scope39/7  "<pq>"
  connections:
  VSI-Droop30/LConn4 -- D-GND30/LConn1
  VSI-Droop31/LConn4 -- D-GND31/LConn1
  VSI-Droop32/LConn4 -- D-GND32/LConn1
  VSI-Droop33/LConn4 -- D-GND33/LConn1
  VSI-Droop34/LConn4 -- D-GND34/LConn1
  VSI-Droop35/LConn4 -- D-GND35/LConn1
  VSI-Droop36/LConn4 -- D-GND36/LConn1
  VSI-Droop37/LConn4 -- D-GND37/LConn1
  VSI-PLL38/LConn4 -- D-GND38/LConn1
  VSI-PLL39/LConn4 -- D-GND39/LConn1
  Branch1-1/RConn1 -- Branch1-1/RConn2 -- Branch1-1/RConn3 -- B-GND1/LConn1
  Branch2-2/RConn1 -- Branch2-2/RConn2 -- Branch2-2/RConn3 -- B-GND4/LConn1
  Branch3-3/RConn1 -- Branch3-3/RConn2 -- Branch3-3/RConn3 -- B-GND9/LConn1
  Branch4-4/RConn1 -- Branch4-4/RConn2 -- Branch4-4/RConn3 -- B-GND12/LConn1
  Branch5-5/RConn1 -- Branch5-5/RConn2 -- Branch5-5/RConn3 -- B-GND15/LConn1
  Branch6-6/RConn1 -- Branch6-6/RConn2 -- Branch6-6/RConn3 -- B-GND18/LConn1
  Branch7-7/RConn1 -- Branch7-7/RConn2 -- Branch7-7/RConn3 -- B-GND22/LConn1
  Branch8-8/RConn1 -- Branch8-8/RConn2 -- Branch8-8/RConn3 -- B-GND24/LConn1
  Branch9-9/RConn1 -- Branch9-9/RConn2 -- Branch9-9/RConn3 -- B-GND26/LConn1
  Branch10-10/RConn1 -- Branch10-10/RConn2 -- Branch10-10/RConn3 -- B-GND27/LConn1
  Branch11-11/RConn1 -- Branch11-11/RConn2 -- Branch11-11/RConn3 -- B-GND31/LConn1
  Branch12-12/RConn1 -- Branch12-12/RConn2 -- Branch12-12/RConn3 -- B-GND33/LConn1
  Branch13-13/RConn1 -- Branch13-13/RConn2 -- Branch13-13/RConn3 -- B-GND35/LConn1
  Branch14-14/RConn1 -- Branch14-14/RConn2 -- Branch14-14/RConn3 -- B-GND37/LConn1
  Branch15-15/RConn1 -- Branch15-15/RConn2 -- Branch15-15/RConn3 -- B-GND39/LConn1
  Branch16-16/RConn1 -- Branch16-16/RConn2 -- Branch16-16/RConn3 -- B-GND41/LConn1
  Branch17-17/RConn1 -- Branch17-17/RConn2 -- Branch17-17/RConn3 -- B-GND46/LConn1
  Branch18-18/RConn1 -- Branch18-18/RConn2 -- Branch18-18/RConn3 -- B-GND49/LConn1
  Branch19-19/RConn1 -- Branch19-19/RConn2 -- Branch19-19/RConn3 -- B-GND50/LConn1
  Branch20-20/RConn1 -- Branch20-20/RConn2 -- Branch20-20/RConn3 -- B-GND53/LConn1
  Branch21-21/RConn1 -- Branch21-21/RConn2 -- Branch21-21/RConn3 -- B-GND55/LConn1
  Branch22-22/RConn1 -- Branch22-22/RConn2 -- Branch22-22/RConn3 -- B-GND57/LConn1
  Branch23-23/RConn1 -- Branch23-23/RConn2 -- Branch23-23/RConn3 -- B-GND60/LConn1
  Branch24-24/RConn1 -- Branch24-24/RConn2 -- Branch24-24/RConn3 -- B-GND63/LConn1
  Branch25-25/RConn1 -- Branch25-25/RConn2 -- Branch25-25/RConn3 -- B-GND64/LConn1
  Branch26-26/RConn1 -- Branch26-26/RConn2 -- Branch26-26/RConn3 -- B-GND67/LConn1
  Branch27-27/RConn1 -- Branch27-27/RConn2 -- Branch27-27/RConn3 -- B-GND71/LConn1
  Branch28-28/RConn1 -- Branch28-28/RConn2 -- Branch28-28/RConn3 -- B-GND72/LConn1
  Branch29-29/RConn1 -- Branch29-29/RConn2 -- Branch29-29/RConn3 -- B-GND74/LConn1
  Branch31-31/RConn1 -- Branch31-31/RConn2 -- Branch31-31/RConn3 -- B-GND76/LConn1
  Branch39-39/RConn1 -- Branch39-39/RConn2 -- Branch39-39/RConn3 -- B-GND77/LConn1
  Branch1-9/RConn1 -- Bus9/RConn1 -- Branch9-9/LConn1 -- Branch8-9/RConn1
  Branch1-9/RConn2 -- Bus9/RConn2 -- Branch9-9/LConn2 -- Branch8-9/RConn2
  Branch1-9/RConn3 -- Bus9/RConn3 -- Branch9-9/LConn3 -- Branch8-9/RConn3
  Branch1-9/LConn1 -- Bus1/RConn1 -- Branch1-1/LConn1 -- Branch1-39/LConn1
  Branch1-9/LConn2 -- Bus1/RConn2 -- Branch1-1/LConn2 -- Branch1-39/LConn2
  Branch1-9/LConn3 -- Bus1/RConn3 -- Branch1-1/LConn3 -- Branch1-39/LConn3
  Branch1-39/RConn1 -- Bus39/RConn1 -- Branch39-39/LConn1 -- Branch2-39/RConn1
  Branch1-39/RConn2 -- Bus39/RConn2 -- Branch39-39/LConn2 -- Branch2-39/RConn2
  Branch1-39/RConn3 -- Bus39/RConn3 -- Branch39-39/LConn3 -- Branch2-39/RConn3
  Branch2-3/RConn1 -- Bus3/RConn1 -- Branch3-3/LConn1 -- Branch3-18/LConn1 -- Branch3-4/LConn1
  Branch2-3/RConn2 -- Bus3/RConn2 -- Branch3-3/LConn2 -- Branch3-18/LConn2 -- Branch3-4/LConn2
  Branch2-3/RConn3 -- Bus3/RConn3 -- Branch3-3/LConn3 -- Branch3-18/LConn3 -- Branch3-4/LConn3
  Branch2-3/LConn1 -- Bus2/RConn1 -- Branch2-2/LConn1 -- Branch2-39/LConn1 -- Transformer2-30/LConn1 -- Branch2-25/LConn1
  Branch2-3/LConn2 -- Bus2/RConn2 -- Branch2-2/LConn2 -- Branch2-39/LConn2 -- Transformer2-30/LConn2 -- Branch2-25/LConn2
  Branch2-3/LConn3 -- Bus2/RConn3 -- Branch2-2/LConn3 -- Branch2-39/LConn3 -- Transformer2-30/LConn3 -- Branch2-25/LConn3
  Branch2-25/RConn1 -- Bus25/RConn1 -- Branch25-25/LConn1 -- Transformer25-37/LConn1 -- Branch25-26/LConn1
  Branch2-25/RConn2 -- Bus25/RConn2 -- Branch25-25/LConn2 -- Transformer25-37/LConn2 -- Branch25-26/LConn2
  Branch2-25/RConn3 -- Bus25/RConn3 -- Branch25-25/LConn3 -- Transformer25-37/LConn3 -- Branch25-26/LConn3
  Bus30/RConn1 -- Branch2-30/RConn1
  Bus30/RConn2 -- Branch2-30/RConn2
  Bus30/RConn3 -- Branch2-30/RConn3
  Transformer2-30/RConn1 -- Branch2-30/LConn1
  Transformer2-30/RConn2 -- Branch2-30/LConn2
  Transformer2-30/RConn3 -- Branch2-30/LConn3
  Branch3-4/RConn1 -- Bus4/RConn1 -- Branch4-4/LConn1 -- Branch4-14/LConn1 -- Branch4-5/LConn1
  Branch3-4/RConn2 -- Bus4/RConn2 -- Branch4-4/LConn2 -- Branch4-14/LConn2 -- Branch4-5/LConn2
  Branch3-4/RConn3 -- Bus4/RConn3 -- Branch4-4/LConn3 -- Branch4-14/LConn3 -- Branch4-5/LConn3
  Branch3-18/RConn1 -- Bus18/RConn1 -- Branch18-18/LConn1 -- Branch17-18/RConn1
  Branch3-18/RConn2 -- Bus18/RConn2 -- Branch18-18/LConn2 -- Branch17-18/RConn2
  Branch3-18/RConn3 -- Bus18/RConn3 -- Branch18-18/LConn3 -- Branch17-18/RConn3
  Branch4-5/RConn1 -- Bus5/RConn1 -- Branch5-5/LConn1 -- Branch5-8/LConn1 -- Branch5-6/LConn1
  Branch4-5/RConn2 -- Bus5/RConn2 -- Branch5-5/LConn2 -- Branch5-8/LConn2 -- Branch5-6/LConn2
  Branch4-5/RConn3 -- Bus5/RConn3 -- Branch5-5/LConn3 -- Branch5-8/LConn3 -- Branch5-6/LConn3
  Branch4-14/RConn1 -- Bus14/RConn1 -- Branch14-14/LConn1 -- Branch14-15/LConn1 -- Branch13-14/RConn1
  Branch4-14/RConn2 -- Bus14/RConn2 -- Branch14-14/LConn2 -- Branch14-15/LConn2 -- Branch13-14/RConn2
  Branch4-14/RConn3 -- Bus14/RConn3 -- Branch14-14/LConn3 -- Branch14-15/LConn3 -- Branch13-14/RConn3
  Branch5-6/RConn1 -- Bus6/RConn1 -- Branch6-6/LConn1 -- Transformer6-31/LConn1 -- Branch6-11/LConn1 -- Branch6-7/LConn1
  Branch5-6/RConn2 -- Bus6/RConn2 -- Branch6-6/LConn2 -- Transformer6-31/LConn2 -- Branch6-11/LConn2 -- Branch6-7/LConn2
  Branch5-6/RConn3 -- Bus6/RConn3 -- Branch6-6/LConn3 -- Transformer6-31/LConn3 -- Branch6-11/LConn3 -- Branch6-7/LConn3
  Branch5-8/RConn1 -- Bus8/RConn1 -- Branch8-8/LConn1 -- Branch8-9/LConn1 -- Branch7-8/RConn1
  Branch5-8/RConn2 -- Bus8/RConn2 -- Branch8-8/LConn2 -- Branch8-9/LConn2 -- Branch7-8/RConn2
  Branch5-8/RConn3 -- Bus8/RConn3 -- Branch8-8/LConn3 -- Branch8-9/LConn3 -- Branch7-8/RConn3
  Branch6-7/RConn1 -- Bus7/RConn1 -- Branch7-7/LConn1 -- Branch7-8/LConn1
  Branch6-7/RConn2 -- Bus7/RConn2 -- Branch7-7/LConn2 -- Branch7-8/LConn2
  Branch6-7/RConn3 -- Bus7/RConn3 -- Branch7-7/LConn3 -- Branch7-8/LConn3
  Branch6-11/RConn1 -- Bus11/RConn1 -- Branch11-11/LConn1 -- Transformer11-12/LConn1 -- Branch10-11/RConn1
  Branch6-11/RConn2 -- Bus11/RConn2 -- Branch11-11/LConn2 -- Transformer11-12/LConn2 -- Branch10-11/RConn2
  Branch6-11/RConn3 -- Bus11/RConn3 -- Branch11-11/LConn3 -- Transformer11-12/LConn3 -- Branch10-11/RConn3
  Branch6-31/RConn1 -- Bus31/RConn1 -- Branch31-31/LConn1
  Branch6-31/RConn2 -- Bus31/RConn2 -- Branch31-31/LConn2
  Branch6-31/RConn3 -- Bus31/RConn3 -- Branch31-31/LConn3
  Transformer6-31/RConn1 -- Branch6-31/LConn1
  Transformer6-31/RConn2 -- Branch6-31/LConn2
  Transformer6-31/RConn3 -- Branch6-31/LConn3
  Branch10-11/LConn1 -- Bus10/RConn1 -- Branch10-10/LConn1 -- Transformer10-32/LConn1 -- Branch10-13/LConn1
  Branch10-11/LConn2 -- Bus10/RConn2 -- Branch10-10/LConn2 -- Transformer10-32/LConn2 -- Branch10-13/LConn2
  Branch10-11/LConn3 -- Bus10/RConn3 -- Branch10-10/LConn3 -- Transformer10-32/LConn3 -- Branch10-13/LConn3
  Branch10-13/RConn1 -- Bus13/RConn1 -- Branch13-13/LConn1 -- Branch13-14/LConn1 -- Branch12-13/RConn1
  Branch10-13/RConn2 -- Bus13/RConn2 -- Branch13-13/LConn2 -- Branch13-14/LConn2 -- Branch12-13/RConn2
  Branch10-13/RConn3 -- Bus13/RConn3 -- Branch13-13/LConn3 -- Branch13-14/LConn3 -- Branch12-13/RConn3
  Bus32/RConn1 -- Branch10-32/RConn1
  Bus32/RConn2 -- Branch10-32/RConn2
  Bus32/RConn3 -- Branch10-32/RConn3
  Transformer10-32/RConn1 -- Branch10-32/LConn1
  Transformer10-32/RConn2 -- Branch10-32/LConn2
  Transformer10-32/RConn3 -- Branch10-32/LConn3
  Branch11-12/RConn1 -- Bus12/RConn1 -- Branch12-12/LConn1 -- Transformer12-13/LConn1
  Branch11-12/RConn2 -- Bus12/RConn2 -- Branch12-12/LConn2 -- Transformer12-13/LConn2
  Branch11-12/RConn3 -- Bus12/RConn3 -- Branch12-12/LConn3 -- Transformer12-13/LConn3
  Transformer11-12/RConn1 -- Branch11-12/LConn1
  Transformer11-12/RConn2 -- Branch11-12/LConn2
  Transformer11-12/RConn3 -- Branch11-12/LConn3
  Transformer12-13/RConn1 -- Branch12-13/LConn1
  Transformer12-13/RConn2 -- Branch12-13/LConn2
  Transformer12-13/RConn3 -- Branch12-13/LConn3
  Branch14-15/RConn1 -- Bus15/RConn1 -- Branch15-15/LConn1 -- Branch15-16/LConn1
  Branch14-15/RConn2 -- Bus15/RConn2 -- Branch15-15/LConn2 -- Branch15-16/LConn2
  Branch14-15/RConn3 -- Bus15/RConn3 -- Branch15-15/LConn3 -- Branch15-16/LConn3
  Branch15-16/RConn1 -- Bus16/RConn1 -- Branch16-16/LConn1 -- Branch16-24/LConn1 -- Branch16-21/LConn1 -- Branch16-19/LConn1 -- Branch16-17/LConn1
  Branch15-16/RConn2 -- Bus16/RConn2 -- Branch16-16/LConn2 -- Branch16-24/LConn2 -- Branch16-21/LConn2 -- Branch16-19/LConn2 -- Branch16-17/LConn2
  Branch15-16/RConn3 -- Bus16/RConn3 -- Branch16-16/LConn3 -- Branch16-24/LConn3 -- Branch16-21/LConn3 -- Branch16-19/LConn3 -- Branch16-17/LConn3
  Branch16-17/RConn1 -- Bus17/RConn1 -- Branch17-17/LConn1 -- Branch17-27/LConn1 -- Branch17-18/LConn1
  Branch16-17/RConn2 -- Bus17/RConn2 -- Branch17-17/LConn2 -- Branch17-27/LConn2 -- Branch17-18/LConn2
  Branch16-17/RConn3 -- Bus17/RConn3 -- Branch17-17/LConn3 -- Branch17-27/LConn3 -- Branch17-18/LConn3
  Branch16-19/RConn1 -- Bus19/RConn1 -- Branch19-19/LConn1 -- Transformer19-33/LConn1 -- Transformer19-20/LConn1
  Branch16-19/RConn2 -- Bus19/RConn2 -- Branch19-19/LConn2 -- Transformer19-33/LConn2 -- Transformer19-20/LConn2
  Branch16-19/RConn3 -- Bus19/RConn3 -- Branch19-19/LConn3 -- Transformer19-33/LConn3 -- Transformer19-20/LConn3
  Branch16-21/RConn1 -- Bus21/RConn1 -- Branch21-21/LConn1 -- Branch21-22/LConn1
  Branch16-21/RConn2 -- Bus21/RConn2 -- Branch21-21/LConn2 -- Branch21-22/LConn2
  Branch16-21/RConn3 -- Bus21/RConn3 -- Branch21-21/LConn3 -- Branch21-22/LConn3
  Branch16-24/RConn1 -- Bus24/RConn1 -- Branch24-24/LConn1 -- Branch23-24/RConn1
  Branch16-24/RConn2 -- Bus24/RConn2 -- Branch24-24/LConn2 -- Branch23-24/RConn2
  Branch16-24/RConn3 -- Bus24/RConn3 -- Branch24-24/LConn3 -- Branch23-24/RConn3
  Branch17-27/RConn1 -- Bus27/RConn1 -- Branch27-27/LConn1 -- Branch26-27/RConn1
  Branch17-27/RConn2 -- Bus27/RConn2 -- Branch27-27/LConn2 -- Branch26-27/RConn2
  Branch17-27/RConn3 -- Bus27/RConn3 -- Branch27-27/LConn3 -- Branch26-27/RConn3
  Branch19-20/RConn1 -- Bus20/RConn1 -- Branch20-20/LConn1 -- Transformer20-34/LConn1
  Branch19-20/RConn2 -- Bus20/RConn2 -- Branch20-20/LConn2 -- Transformer20-34/LConn2
  Branch19-20/RConn3 -- Bus20/RConn3 -- Branch20-20/LConn3 -- Transformer20-34/LConn3
  Transformer19-20/RConn1 -- Branch19-20/LConn1
  Transformer19-20/RConn2 -- Branch19-20/LConn2
  Transformer19-20/RConn3 -- Branch19-20/LConn3
  Bus33/RConn1 -- Branch19-33/RConn1
  Bus33/RConn2 -- Branch19-33/RConn2
  Bus33/RConn3 -- Branch19-33/RConn3
  Transformer19-33/RConn1 -- Branch19-33/LConn1
  Transformer19-33/RConn2 -- Branch19-33/LConn2
  Transformer19-33/RConn3 -- Branch19-33/LConn3
  Bus34/RConn1 -- Branch20-34/RConn1
  Bus34/RConn2 -- Branch20-34/RConn2
  Bus34/RConn3 -- Branch20-34/RConn3
  Transformer20-34/RConn1 -- Branch20-34/LConn1
  Transformer20-34/RConn2 -- Branch20-34/LConn2
  Transformer20-34/RConn3 -- Branch20-34/LConn3
  Branch21-22/RConn1 -- Bus22/RConn1 -- Branch22-22/LConn1 -- Transformer22-35/LConn1 -- Branch22-23/LConn1
  Branch21-22/RConn2 -- Bus22/RConn2 -- Branch22-22/LConn2 -- Transformer22-35/LConn2 -- Branch22-23/LConn2
  Branch21-22/RConn3 -- Bus22/RConn3 -- Branch22-22/LConn3 -- Transformer22-35/LConn3 -- Branch22-23/LConn3
  Branch22-23/RConn1 -- Bus23/RConn1 -- Branch23-23/LConn1 -- Branch23-36/LConn1 -- Branch23-24/LConn1
  Branch22-23/RConn2 -- Bus23/RConn2 -- Branch23-23/LConn2 -- Branch23-36/LConn2 -- Branch23-24/LConn2
  Branch22-23/RConn3 -- Bus23/RConn3 -- Branch23-23/LConn3 -- Branch23-36/LConn3 -- Branch23-24/LConn3
  Bus35/RConn1 -- Branch22-35/RConn1
  Bus35/RConn2 -- Branch22-35/RConn2
  Bus35/RConn3 -- Branch22-35/RConn3
  Transformer22-35/RConn1 -- Branch22-35/LConn1
  Transformer22-35/RConn2 -- Branch22-35/LConn2
  Transformer22-35/RConn3 -- Branch22-35/LConn3
  Bus36/RConn1 -- Branch23-36/RConn1
  Bus36/RConn2 -- Branch23-36/RConn2
  Bus36/RConn3 -- Branch23-36/RConn3
  Branch25-26/RConn1 -- Bus26/RConn1 -- Branch26-26/LConn1 -- Branch26-29/LConn1 -- Branch26-28/LConn1 -- Branch26-27/LConn1
  Branch25-26/RConn2 -- Bus26/RConn2 -- Branch26-26/LConn2 -- Branch26-29/LConn2 -- Branch26-28/LConn2 -- Branch26-27/LConn2
  Branch25-26/RConn3 -- Bus26/RConn3 -- Branch26-26/LConn3 -- Branch26-29/LConn3 -- Branch26-28/LConn3 -- Branch26-27/LConn3
  Bus37/RConn1 -- Branch25-37/RConn1
  Bus37/RConn2 -- Branch25-37/RConn2
  Bus37/RConn3 -- Branch25-37/RConn3
  Transformer25-37/RConn1 -- Branch25-37/LConn1
  Transformer25-37/RConn2 -- Branch25-37/LConn2
  Transformer25-37/RConn3 -- Branch25-37/LConn3
  Branch26-28/RConn1 -- Bus28/RConn1 -- Branch28-28/LConn1 -- Branch28-29/LConn1
  Branch26-28/RConn2 -- Bus28/RConn2 -- Branch28-28/LConn2 -- Branch28-29/LConn2
  Branch26-28/RConn3 -- Bus28/RConn3 -- Branch28-28/LConn3 -- Branch28-29/LConn3
  Branch26-29/RConn1 -- Bus29/RConn1 -- Branch29-29/LConn1 -- Transformer29-38/LConn1 -- Branch28-29/RConn1
  Branch26-29/RConn2 -- Bus29/RConn2 -- Branch29-29/LConn2 -- Transformer29-38/LConn2 -- Branch28-29/RConn2
  Branch26-29/RConn3 -- Bus29/RConn3 -- Branch29-29/LConn3 -- Transformer29-38/LConn3 -- Branch28-29/RConn3
  Bus38/RConn1 -- Branch29-38/RConn1
  Bus38/RConn2 -- Branch29-38/RConn2
  Bus38/RConn3 -- Branch29-38/RConn3
  Transformer29-38/RConn1 -- Branch29-38/LConn1
  Transformer29-38/RConn2 -- Branch29-38/LConn2
  Transformer29-38/RConn3 -- Branch29-38/LConn3
  VSI-Droop30/LConn1 -- Bus30/LConn1
  VSI-Droop30/LConn2 -- Bus30/LConn2
  VSI-Droop30/LConn3 -- Bus30/LConn3
  VSI-Droop31/LConn1 -- Bus31/LConn1
  VSI-Droop31/LConn2 -- Bus31/LConn2
  VSI-Droop31/LConn3 -- Bus31/LConn3
  VSI-Droop32/LConn1 -- Bus32/LConn1
  VSI-Droop32/LConn2 -- Bus32/LConn2
  VSI-Droop32/LConn3 -- Bus32/LConn3
  VSI-Droop33/LConn1 -- Bus33/LConn1
  VSI-Droop33/LConn2 -- Bus33/LConn2
  VSI-Droop33/LConn3 -- Bus33/LConn3
  VSI-Droop34/LConn1 -- Bus34/LConn1
  VSI-Droop34/LConn2 -- Bus34/LConn2
  VSI-Droop34/LConn3 -- Bus34/LConn3
  VSI-Droop35/LConn1 -- Bus35/LConn1
  VSI-Droop35/LConn2 -- Bus35/LConn2
  VSI-Droop35/LConn3 -- Bus35/LConn3
  VSI-Droop36/LConn1 -- Bus36/LConn1
  VSI-Droop36/LConn2 -- Bus36/LConn2
  VSI-Droop36/LConn3 -- Bus36/LConn3
  VSI-Droop37/LConn1 -- Bus37/LConn1
  VSI-Droop37/LConn2 -- Bus37/LConn2
  VSI-Droop37/LConn3 -- Bus37/LConn3
  VSI-PLL38/LConn1 -- Bus38/LConn1
  VSI-PLL38/LConn2 -- Bus38/LConn2
  VSI-PLL38/LConn3 -- Bus38/LConn3
  VSI-PLL39/LConn1 -- Bus39/LConn1
  VSI-PLL39/LConn2 -- Bus39/LConn2
  VSI-PLL39/LConn3 -- Bus39/LConn3
